simulink model "d_3_model"  (Simulink 10.0)
settings: Solver=VariableStepAuto  StartTime=0.0  StopTime=30.0  RelTol=1e-3
settings Model: Creator=aravind  LastModifiedBy=aravind
settings DataIOCC: SaveFormat=Dataset  ReturnWorkspaceOutputs=on
settings OptimizationCC: LifeSpan=auto
settings DebuggingCC: UnderspecifiedInitializationDetection=Simplified  MergeDetectMultiDrivingBlocksExec=error  SFUnexpectedBacktrackingDiag=error  SFNoUnconditionalDefaultTransitionDiag=error  SFExecutionAtInitializationDiag=warning  ArithmeticOperatorsInVariantConditions=error
settings HardwareCC: ProdBitPerPointer=64  ProdBitPerSizeT=64  ProdBitPerPtrDiffT=64  ProdLargestAtomicFloat=Float  ProdIntDivRoundTo=Zero  ProdEndianess=LittleEndian  ProdWordSize=64  ProdHWDeviceType=Intel->x86-64 (Windows64)
settings ModelReferenceCC: PropagateSignalLabelsOutOfModel=on
settings SFSimCC: SimUseLocalCustomCode=on  CustomCodeUndefinedFunction=FilterOut
settings RTWCC: RTWUseLocalCustomCode=on
settings CodeAppCC: StateflowObjectComments=off
settings GRTTargetCC: TargetLangStandard=C99 (ISO)  CombineOutputUpdateFcns=on  GRTInterface=off
settings ConfigComp: CovMetricSettings=dwe  CovHtmlReporting=off  CovSaveCumulativeToWorkspaceVar=off  CovSaveSingleToWorkspaceVar=off

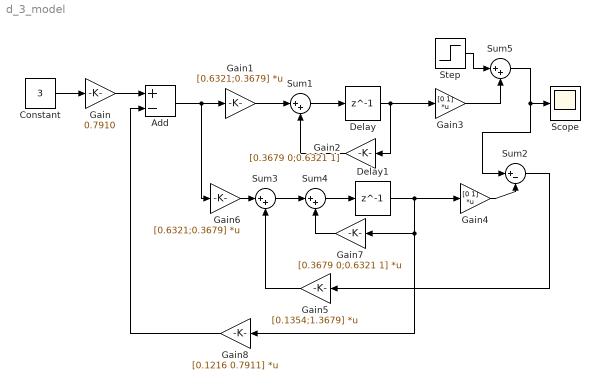
== system d_3_model ==
  Add : Sum  Inputs=+-
  Constant : Constant  Value=3
  Delay : Delay  DelayLength=1  InitialCondition=0
  Delay1 : Delay  DelayLength=1  InitialCondition=0
  Gain : Gain  Gain=0.7910
  Gain1 : Gain  Gain=[0.6321;0.3679]  Multiplication=Matrix(K*u)
  Gain2 : Gain  Gain=[0.3679 0;0.6321 1]
  Gain3 : Gain  Gain=[0 1]  Multiplication=Matrix(K*u)
  Gain4 : Gain  Gain=[0 1]  Multiplication=Matrix(K*u)
  Gain5 : Gain  Gain=[0.1354;1.3679]  Multiplication=Matrix(K*u)
  Gain6 : Gain  Gain=[0.6321;0.3679]  Multiplication=Matrix(K*u)
  Gain7 : Gain  Gain=[0.3679 0;0.6321 1]  Multiplication=Matrix(K*u)
  Gain8 : Gain  Gain=[0.1216 0.7911]  Multiplication=Matrix(K*u)
  Scope : Scope
  Step : Step  Time=0  SampleTime=0
  Sum{1,3..5} (4 alike) : Sum  Inputs=|++
  Sum2 : Sum  Inputs=|+-
  wires:
  Add/1 -> Gain1/1, Gain6/1
  Gain/1 -> Add/1
  Constant/1 -> Gain/1
  Sum1/1 -> Delay/1
  Delay/1 -> Gain3/1, Gain2/1
  Gain2/1 -> Sum1/2
  Gain1/1 -> Sum1/1
  Gain4/1 -> Sum2/2
  Sum2/1 -> Gain5/1
  Gain5/1 -> Sum3/2
  Gain6/1 -> Sum3/1
  Sum4/1 -> Delay1/1
  Sum3/1 -> Sum4/1
  Gain7/1 -> Sum4/2
  Delay1/1 -> Gain8/1, Gain7/1, Gain4/1
  Gain8/1 -> Add/2
  Step/1 -> Sum5/1
  Gain3/1 -> Sum5/2
  Sum5/1 -> Sum2/1, Scope/1
